simulink model "windEmulatorStep4"  (R2025b)
settings: Solver=ode4  StartTime=0.0  StopTime=inf  FixedStep=Ts  RelTol=1e-3
values from neighbouring files (symbols this model uses):
  A = 1.0    (= 1)    [initStep4.m]
  absEncoderCountsToRad = 1/2^20*2*pi    (= 5.99211245268e-06)    [initStep4.m]
  acs800CtrlStruct =     [windEmulatorBusDefs.mat]
  acs800DcBusVoltsScaling = 1    [initStep4.m]
  acs800FreqScaling = 1/100    (= 0.01)    [initStep4.m]
  acs800PowerScaling = Gen_PowerScaling    (= 14.9109)    [initStep4.m]
  acs800SignalStruct =     [windEmulatorBusDefs.mat]
  acs800SpeedNomEng = 1500    [initStep4.m]
  acs800SpeedNomFb = 20000    [initStep4.m]
  acs800SpeedScaling = 1500/20000    (= 0.075)    [initStep4.m]
  acs800TempScaling = 1/10    (= 0.1)    [initStep4.m]
  acs800TorqueNomEng = 100    [initStep4.m]
  acs800TorqueNomFb = 10000    [initStep4.m]
  acs800TorqueScaling = acs800TorqueRating/10000    (= 0.008035933)    [initStep4.m]
  acs880CtrlStruct =     [windEmulatorBusDefs.mat]
  acs880FreqScaling = 60/20000    (= 0.003)    [initStep4.m]
  acs880MotorCurrentScaling = 100/10000    (= 0.01)    [initStep4.m]
  acs880MotorVoltsScaling = 1    [initStep4.m]
  acs880PowerScaling = 100*hp2W/10000    (= 7.457)    [initStep4.m]
  acs880RatedTorque = 80.494    [initStep4.m]
  acs880RateLimFalling = -10000    [initStep4.m]
  acs880RateLimRising = 10000    [initStep4.m]
  acs880SetpointLimLower = -0.975*acs880RatedTorque    (= -78.48165)    [initStep4.m]
  acs880SetpointLimUpper = 0.975*acs880RatedTorque    (= 78.48165)    [initStep4.m]
  acs880SignalStruct =     [windEmulatorBusDefs.mat]
  acs880SpeedPILimLo = -0.975*acs880RatedTorque    (= -78.48165)    [initStep4.m]
  acs880SpeedPILimUp = 0.975*acs880RatedTorque    (= 78.48165)    [initStep4.m]
  acs880SpeedScaling = 2000/20000    (= 0.1)    [initStep4.m]
  acs880TorqueFieldbusScale = 10000    [initStep4.m]
  acs880TorqueScaling = acs880RatedTorque/acs880TorqueFieldbusScale    (= 0.0080494)    [initStep4.m]
  acs880TorqueSetpointScaling = 100    [initStep4.m]
  bar2pa = 1e5    (= 100000)    [initStep4.m]
  belowMinPGain = 1/200    (= 0.005)    [initStep4.m]
  ctrlModeTorque = logical(true)    [init.m]    (also in initStep1.m; initStep2.m; initStep3.m; initStep4.m)
  ctrlSignal1 = squeeze(hptoSignalsData.Values.ctrlSignal1.Data)    [postProcessingStep2.m]
  ctrlSignal2 = squeeze(hptoSignalsData.Values.ctrlSignal2.Data)    [postProcessingStep2.m]
  deadBandController = boolean(false)    [initStep4.m]
  deadbandTorqueSlewRate = 300    [initStep4.m]
  Dm_max = 40    [initStep4.m]
  EffMechMax = 0.93    [initStep4.m]
  EffMechMin = 0.79    [initStep4.m]
  excForce_N = squeeze(hptoCtrlData.Values.excForce_N.Data)    [postProcessingStep2.m]
  expCtrlStruct =     [windEmulatorBusDefs.mat]
  FactorEff = psi2pa*cc2m3*(1/rev2rad)    (= 0.00109733470463)    [initStep4.m]
  fromFileSpeedSlewRate = 250    [initStep4.m]
  fromFileTorqueSlewRate = 25    [initStep4.m]
  futekTorqueScale = -1/(2^31)*10/5*100    (= -9.31322574615e-08)    [initStep4.m]
  genMaxTorque = 0.8*ratedTorque    (= 64.3952)    [initStep3.m]    (also in initStep4.m = 78.48165)
  genTorqueCmd_Nm = squeeze(hptoSignalsData.Values.genTorqueCmd_Nm.Data)    [postProcessingStep2.m]
  hbmCtScale = 1/1.5    (= 0.666666666667)    [initStep4.m]
  hbmPowerStruct =     [windEmulatorBusDefs.mat]
  hptoCtrlStruct =     [windEmulatorBusDefs.mat]
  hptoSignalStruct =     [windEmulatorBusDefs.mat]
  invPowerStruct =     [windEmulatorBusDefs.mat]
  lpm2m3ps = 1/m3ps2lpm    (= 1.66666666667e-05)    [initStep4.m]
  minPressureRef_psi = 1000    [initStep4.m]
  minTorqueRef_Nm = (minPressureRef_psi*psi2pa)*(Dm_max*cc2m3*(1/rev2rad))    (= 43.8933881851)    [initStep4.m]
  motorSpeed_rpm = squeeze(acs880SignalsData.Values.motorSpeed_rpm.Data)    [postProcessingStep2.m]
  nPreDrop = 2900    [initStep4.m]
  nPreDropMin = 725    [initStep4.m]
  psi2bar = 1/bar2psi    (= 0.0689475729318)    [initStep4.m]
  radps2rpm = 60/(2*pi)    (= 9.54929658551)    [initStep2.m]    (also in initStep4.m)
  rpm2radps = 2*pi/60    (= 0.10471975512)    [initStep4.m]
  runCounter = squeeze(hptoCtrlData.Values.runCounter.Data)    [postProcessingStep2.m]
  shaftSignalStruct =     [windEmulatorBusDefs.mat]
  sidCtrlStruct =     [windEmulatorBusDefs.mat]
  sidDataCaseCounter = sidData.experimentData.count    [initStep4.m]
  sidDataSpeed_rpm = sidData.experimentData.wShaft_rpm    [initStep4.m]
  sidDataTorque_Nm = sidData.experimentData.torqueShaft_Nm    [initStep4.m]
  sidInfoStruct =     [windEmulatorBusDefs.mat]
  T = 4    [initStep4.m]
  targetOmega = 2000/60*2*pi    (= 209.439510239)    [initStep2.m]    (also in initStep3.m; initStep4.m)
  time = hptoCtrlData.Values.runCounter.Time    [postProcessingStep2.m]
  TorqueLoadMax = 75    [initStep4.m]
  Ts = 1/250    (= 0.004)    [initStep4.m]
undefined symbols (not defined in the file or in its folder): absEncoderCounts, absEncoderPosition_rad, absEncoderSpeed_rpm, absEncoderStatus1, absEncoderStatus2, absEncoderTurns, acs800Torque_Nm, acs800TorqueSetpoint_Nm, acs880SpeedSetpoint_rpm, acs880Torque_Nm, ctrlWord, dcBusVoltage_V, DiscIntNeverNeededParam, excShaftSpeed_rpm, excShaftTorque_Nm, expType, expTypeEnum, frequency_Hz, fromFileCaseCounter, genPumpFlow_lpm, genShaftSpeed_rpm, genSpeedActual, hmOutputShafTorque_Nm, motorCurrent_A, motorTorque_Nm, motorVoltage_V, pressure_bar, PressureControl, ramp, resetHilIntegrator, resetSidIntegrator, runHil, runSid, shaftPower_W, sidType, sidTypeEnum, SpeedControl, speedCtrlReset, speedRef_rpm, state, statusWord, stepCounter, temperature, torqueActual_Nm, TorqueInputControl, torqueSetpoint_Nm, torqueSetpoint_percent
libraries: slrealtimeethercatlib x118, fl_lib x26, nesl_utility x17, slrealtimeloglib x13, sh_lib x9, dspstat3 x5, simulink_extras x4, slpidlib x3, cstblocks x3, dspindex x3, simulink x2
(part 4 of 5)

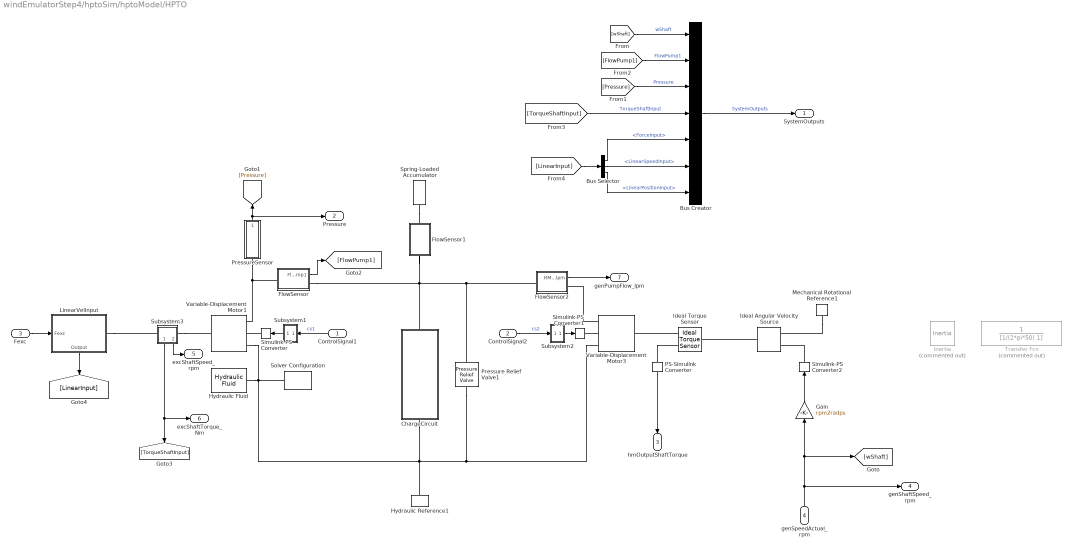
== system windEmulatorStep4/hptoSim/hptoModel/HPTO ==
  ControlSignal1 : Inport
  ControlSignal2 : Inport  Port=2
  Fexc : Inport  Port=3
  genSpeedActual_rpm : Inport  Port=4
  Bus Creator : BusCreator  Inputs=7
  Bus Selector : BusSelector  OutputSignals=ForceInput,LinearSpeedInput,LinearPositionInput
  ChargeCircuit : Subsystem
  FlowSensor : Subsystem
  FlowSensor1 : Subsystem
  FlowSensor2 : Subsystem
  Gain : Gain  Gain=rpm2radps
  Hydraulic Fluid : sh_lib/Hydraulic Utilities/Hydraulic Fluid  SelFluid=1  SysTemp=60  TrapAir=0.005  ViscDerFactor=1  range_error=1  suppress_warning=false
  Hydraulic Reference1 : fl_lib/Hydraulic/Hydraulic Elements/Hydraulic Reference
  Ideal Angular Velocity Source : fl_lib/Mechanical/Mechanical Sources/Ideal Angular Velocity Source
  Ideal Torque Sensor : fl_lib/Mechanical/Mechanical Sensors/Ideal Torque Sensor
  Inertia : fl_lib/Mechanical/Rotational Elements/Inertia  Commented=on  inertia=genShaftInertia_kgm2 kg*m^2  num_ports=foundation.enum.numPorts2.one  w_specify=off  w_priority=High  w=0 rad/s  w_nominal_specify=off  w_nominal_value=1  w_nominal_unit=rad/s  t_specify=off  t_priority=None  t=0 N*m  t_nominal_specify=off  t_nominal_value=1  t_nominal_unit=N*m
  LinearVelInput : Subsystem
      settings: PortSchema="{\"entries\":[{\"content\":{\"sides\":[{\"content\":{\"connectorIds\":[\"LConn1\"]},\"type\":\"ConnectorPlacement.EquallySpacedRectSide\",\"uuid\":\"4859a0f7-9f9b-474b-bb49-bd256c408622\"},{\"content\":{\"connectorIds\":[\"In1\"],\"side\":\"RIGHT\"},\"type\":\"ConnectorPlacement.EquallySpacedRectSide\",\"uuid\":\"5e25e59b-8f8b-4773-b6d9-951d4129523a\"},{\"content\":{\"connectorIds\":[],\"side\":\"TOP\"},\"type\":\"ConnectorPlacement.EquallySpacedRectSide\",\"uuid\":\"bae24e3d-e286-4bf4-a21b-122b1e5bc09f\"},{\"content\":{\"connectorIds\":[\"Out1\"],\"side\":\"BOTTOM\"},\"type\":\"ConnectorPlacement.EquallySpacedRectSide\",\"uuid\":\"0ce66b8b-3f3a-4f1a-9606-df56b31d9b3c\"}]},\"type\":\"ConnectorPlacement.EquallySpacedConnector\",\"uuid\":\"f87c39b6-c8d4-4afb-9096-6dab01ec5afa\"}],\"packageUris\":[\"http://schema.mathworks.com/mf0/Connector/R2020b\"],\"version\":\"1.0\"}"
  Mechanical Rotational Reference1 : fl_lib/Mechanical/Rotational Elements/Mechanical Rotational Reference
  PS-Simulink Converter : nesl_utility/PS-Simulink Converter  PhysicalDomain=network_engine_domain  SubClassName=ps_output  LeftPortType=input  RightPortType=output  PseudoPeriodic=off  Frequencies=[]  VectorFormat=1-D array  Unit=inherit  AffineConversion=off
  Pressure Relief Valve1 : sh_lib/Valves/Pressure Control Valves/Pressure Relief Valve  valve_area_spec=1  p_diff_TLU=[30.15e5 : 15e3 : 31.35e5] Pa  area_TLU=[1 : 1 : 9] .* 1e-5 m^2  area_max=(3.557e-4) m^2  pres_set=PressureValveMax psi  reg_range=ValvePreRange psi  C_d=0.7  A_leak=1e-12 m^2  lam_spec=1  B_lam=0.999  Re_cr=12  dynamic=0  tau=0.1 s  area_init=1e-12 m^2
      settings: InternalSimscapePortConfiguration="{\"Bottom\":[],\"Left\":[{\"id\":\"A\",\"label\":\"A\",\"type\":\"foundation.hydraulic.hydraulic\"}],\"Right\":[{\"id\":\"B\",\"label\":\"B\",\"type\":\"foundation.hydraulic.hydraulic\"}],\"Top\":[]}"
  PressureSensor : Subsystem
  Simulink-PS Converter : nesl_utility/Simulink-PS Converter  PhysicalDomain=network_engine_domain  SubClassName=ps_input  LeftPortType=input  RightPortType=output  PseudoPeriodic=off  Frequencies=[]  NoiseDistribution=none  NoiseParameters=[]  Unit=1  AffineConversion=off  FilteringAndDerivatives=provide  SimscapeFilterOrder=1  InputFilterTimeConstant=0.001  UdotUserProvided=0
  Simulink-PS Converter1 : nesl_utility/Simulink-PS Converter  PhysicalDomain=network_engine_domain  SubClassName=ps_input  LeftPortType=input  RightPortType=output  PseudoPeriodic=off  Frequencies=[]  NoiseDistribution=none  NoiseParameters=[]  Unit=1  AffineConversion=off  FilteringAndDerivatives=provide  SimscapeFilterOrder=1  InputFilterTimeConstant=0.001  UdotUserProvided=0
  Simulink-PS Converter2 : nesl_utility/Simulink-PS Converter  PhysicalDomain=network_engine_domain  SubClassName=ps_input  LeftPortType=input  RightPortType=output  PseudoPeriodic=off  Frequencies=[]  NoiseDistribution=none  NoiseParameters=[]  Unit=1  AffineConversion=off  FilteringAndDerivatives=provide  SimscapeFilterOrder=1  InputFilterTimeConstant=0.001  UdotUserProvided=0
  Solver Configuration : nesl_utility/Solver Configuration  PhysicalDomain=network_engine_domain  SubClassName=solver  LeftPortType=input  RightPortType=generic  Tones=[]  Harmonics=[]  SimulateNoise=off  Profile=off  UseLocalSampling=off  EnableSwitchedLinearOptims=on  FrequencyDomain=off  UseCCode=off  RelTol=0.001  AbsTol=1e-06  MinStep=1e-09  ToWorkspace=off  RevertToSquareIcSolve=off  NumHomotopyIterations=100  PhasorMode=off  PhasorModeNumHarmonics=1  ConsistencySolver=NEWTON_FTOL  IndexReductionMethod=DerivativeReplacement  DoDC=off  ResidualTolerance=1e-09  ConsistencyTolSource=GLOBAL  ConsistencyAbsTol=0.001  ConsistencyRelTol=0.001  ConsistencyTolFactor=0.001  UseLocalSolver=on  LocalSolverChoice=NE_BACKWARD_EULER_ADVANCER  ResolveIndetEquations=on  FunctionEvalNumThread=1  LocalSolverSampleTime=Ts  DoFixedCost=on  MaxNonlinIter=3  MaxModeIter=2  ComputeImpulses=off  ImpulseIterations=2  LinearAlgebra=auto  LinearAlgebraNumThread=0  EquationFormulation=NE_TIME_EF  DelaysMemoryBudget=1024  AutomaticFiltering=on  FilteringTimeConstant=0.001  PartitionStorageMethod=AS_NEEDED  PartitionMemoryBudget=1024  PartitionMethod=ROBUST  MultibodyUseLocalSolver=off  MultibodyLocalSolverChoice=ODE1  MultibodyLocalSolverSampleTime=0.001
  Spring-Loaded Accumulator : sh_lib/Accumulators/Spring-Loaded Accumulator  capacity=AccVol m^3  pr_preload=Acc_PC psi  pr_max=Acc_MaxP psi  stiff_coeff=1e10 Pa/m^3  penetr_coeff=1e10 Pa*s/m^6  flow_rate_specify=off  flow_rate_priority=None  flow_rate=5e-3 m^3/s  flow_rate_nominal_specify=off  flow_rate_nominal_value=1  flow_rate_nominal_unit=m^3/s  fluid_volume_specify=on  fluid_volume_priority=None  fluid_volume=5e-6 m^3  fluid_volume_nominal_specify=off  fluid_volume_nominal_value=1  fluid_volume_nominal_unit=m^3  fluid_pressure_specify=off  fluid_pressure_priority=None  fluid_pressure=1.01325e5 Pa  fluid_pressure_nominal_specify=off  fluid_pressure_nominal_value=1  fluid_pressure_nominal_unit=Pa
      settings: InternalSimscapePortConfiguration="{\"Bottom\":[],\"Left\":[],\"Right\":[{\"id\":\"A\",\"label\":\"A\",\"type\":\"foundation.hydraulic.hydraulic\"}],\"Top\":[]}"
  Subsystem1 : Subsystem
  Subsystem2 : Subsystem
  Subsystem3 : Subsystem
      settings: PortSchema="{\"entries\":[{\"content\":{\"sides\":[{\"content\":{\"connectorIds\":[\"LConn1\"]},\"type\":\"ConnectorPlacement.EquallySpacedRectSide\",\"uuid\":\"7d5827d5-19d2-449a-bfe5-3899d5f2f234\"},{\"content\":{\"connectorIds\":[\"RConn1\"],\"side\":\"RIGHT\"},\"type\":\"ConnectorPlacement.EquallySpacedRectSide\",\"uuid\":\"27ad7fb5-d235-43aa-a783-09c3ddbf3629\"},{\"content\":{\"connectorIds\":[],\"side\":\"TOP\"},\"type\":\"ConnectorPlacement.EquallySpacedRectSide\",\"uuid\":\"41db419c-7193-454e-a54e-cfb74ab94a84\"},{\"content\":{\"connectorIds\":[\"Out1\",\"Out2\"],\"side\":\"BOTTOM\"},\"type\":\"ConnectorPlacement.EquallySpacedRectSide\",\"uuid\":\"63d69fbc-18e5-4f7b-99db-9fcc8740eddf\"}]},\"type\":\"ConnectorPlacement.EquallySpacedConnector\",\"uuid\":\"1d29a5fa-8394-444f-93a2-8698ce035363\"}],\"packageUris\":[\"http://schema.mathworks.com/mf0/Connector/R2020b\"],\"version\":\"1.0\"}"
  Transfer Fcn : TransferFcn  Commented=on  Denominator=[1/(2*pi*50) 1]
  Variable-Displacement Motor1 : sh_lib/Pumps and Motors/Variable-Displacement Motor  mdl_type=2  stroke_max=0.005 m  D_max=Dm_max cm^3/rev  cntrl_mem_tab=[-.0075, 0, .0075] m  displ_tab=[-Dm_max, 0, Dm_max] cm^3/rev  interp_method=1  extrap_method=1  loss_spec=1  w_nominal=nShaftSpeed rpm  pr_nominal=nPreDrop psi  visc_nominal=18 cSt  dens_nominal=900 kg/m^3  efficiency_vol=EffVolNom  no_load_torque=nTorqueNoLoad N*m  torque_pressure_coeff=(1/((200-50)*1e5))*Dm_max*FactorEff*((1-EffMechMax)*nPreDrop-(1-EffMechMin)*nPreDropMin) N*m/Pa  p_diff_eff_TLU=[100000, 1000000, 2000000] Pa  omega_eff_TLU=[25, 50, 100, 200, 300, 400] rad/s  displacement_eff_TLU=[-30, -19, 19, 30] cm^3/rev  vol_eff_TLU=repmat([.816, .908, .954, .977, .981, .984; .325, .663, .831, .916, .925, .946; .137, .568, .78, .892, .893, .91], 1, 1, 4)  mech_eff_TLU=repmat([.996, .996, .996, .996, .996, .996; .988, .989, .989, .989, .989, .99; .981, .981, .982, .982, .983, .984], 1, 1, 4)  p_diff_loss_TLU=[100000, 1000000, 2000000] Pa  omega_loss_TLU=[25, 50, 100, 200, 300, 400] rad/s  displacement_loss_TLU=[-30, -19, 19, 30] cm^3/rev  vol_loss_TLU=repmat([.0282, .0253, .0241, .0235, .0291, .0325; .2596, .1271, .1017, .0917, .1216, .1142; .7874, .1901, .141, .1211, .1797, .1978] * 1e-3, 1, 1, 4) m^3/s  mech_loss_TLU=repmat([.002, .002, .002, .002, .002, .002; .06, .055, .055, .055, .055, .05; .19, .19, .18, .18, .17, .16], 1, 1, 4) N*m  pressure_threshold=1e5 Pa  omega_threshold=10 rad/s  displacement_threshold=0.0001 cm^3/rev  octant_check=0  pressure_check=0  min_valid_pressure=0 Pa  vol_eff_min=1e-3  vol_eff_max=1  mech_eff_min=1e-3  mech_eff_max=1
      settings: InternalSimscapePortConfiguration="{\"Bottom\":[],\"Left\":[{\"id\":\"A\",\"label\":\"A\",\"type\":\"foundation.hydraulic.hydraulic\"},{\"id\":\"C\",\"label\":\"C\",\"type\":\"input\"},{\"id\":\"B\",\"label\":\"B\",\"type\":\"foundation.hydraulic.hydraulic\"}],\"Right\":[{\"id\":\"S\",\"label\":\"S\",\"type\":\"foundation.mechanical.rotational.rotational\"}],\"Top\":[]}"
  Variable-Displacement Motor3 : sh_lib/Pumps and Motors/Variable-Displacement Motor  mdl_type=2  stroke_max=0.005 m  D_max=Dm_max cm^3/rev  cntrl_mem_tab=[-.0075, 0, .0075] m  displ_tab=[-Dm_max, 0, Dm_max] cm^3/rev  interp_method=1  extrap_method=1  loss_spec=1  w_nominal=nShaftSpeed rpm  pr_nominal=nPreDrop psi  visc_nominal=18 cSt  dens_nominal=900 kg/m^3  efficiency_vol=EffVolNom  no_load_torque=nTorqueNoLoad N*m  torque_pressure_coeff=(1/((200-50)*1e5))*Dm_max*FactorEff*((1-EffMechMax)*nPreDrop-(1-EffMechMin)*nPreDropMin) N*m/Pa  p_diff_eff_TLU=[100000, 1000000, 2000000] Pa  omega_eff_TLU=[25, 50, 100, 200, 300, 400] rad/s  displacement_eff_TLU=[-30, -19, 19, 30] cm^3/rev  vol_eff_TLU=repmat([.816, .908, .954, .977, .981, .984; .325, .663, .831, .916, .925, .946; .137, .568, .78, .892, .893, .91], 1, 1, 4)  mech_eff_TLU=repmat([.996, .996, .996, .996, .996, .996; .988, .989, .989, .989, .989, .99; .981, .981, .982, .982, .983, .984], 1, 1, 4)  p_diff_loss_TLU=[100000, 1000000, 2000000] Pa  omega_loss_TLU=[25, 50, 100, 200, 300, 400] rad/s  displacement_loss_TLU=[-30, -19, 19, 30] cm^3/rev  vol_loss_TLU=repmat([.0282, .0253, .0241, .0235, .0291, .0325; .2596, .1271, .1017, .0917, .1216, .1142; .7874, .1901, .141, .1211, .1797, .1978] * 1e-3, 1, 1, 4) m^3/s  mech_loss_TLU=repmat([.002, .002, .002, .002, .002, .002; .06, .055, .055, .055, .055, .05; .19, .19, .18, .18, .17, .16], 1, 1, 4) N*m  pressure_threshold=1e5 Pa  omega_threshold=10 rad/s  displacement_threshold=0.00001 cm^3/rev  octant_check=0  pressure_check=0  min_valid_pressure=0 Pa  vol_eff_min=1e-3  vol_eff_max=1  mech_eff_min=1e-3  mech_eff_max=1
      settings: InternalSimscapePortConfiguration="{\"Bottom\":[],\"Left\":[{\"id\":\"A\",\"label\":\"A\",\"type\":\"foundation.hydraulic.hydraulic\"},{\"id\":\"C\",\"label\":\"C\",\"type\":\"input\"},{\"id\":\"B\",\"label\":\"B\",\"type\":\"foundation.hydraulic.hydraulic\"}],\"Right\":[{\"id\":\"S\",\"label\":\"S\",\"type\":\"foundation.mechanical.rotational.rotational\"}],\"Top\":[]}"
  SystemOutputs : Outport
  Pressure : Outport  Port=2
  hmOutputShaftTorque : Outport  Port=3
  genShaftSpeed_rpm : Outport  Port=4
  excShaftSpeed_rpm : Outport  Port=5
  excShaftTorque_Nm : Outport  Port=6
  genPumpFlow_lpm : Outport  Port=7
  wires:
  [wShaft] -> Bus Creator/1  "wShaft"
  PressureSensor/1(Pressure) -> Pressure/1, [Pressure]
  Bus Creator/1 -> SystemOutputs/1  "SystemOutputs"
  ControlSignal1/1 -> Subsystem1/1(In1)  "cs1"
  Subsystem1/1(Out1) -> Simulink-PS Converter/1
  Subsystem2/1(Out1) -> Simulink-PS Converter1/1
  ControlSignal2/1 -> Subsystem2/1(1)  "cs2"
  FlowSensor/1(FlowPump1) -> [FlowPump1]
  [FlowPump1] -> Bus Creator/2  "FlowPump1"
  [Pressure] -> Bus Creator/3  "Pressure"
  Subsystem3/1(torque_Nm) -> excShaftTorque_Nm/1, [TorqueShaftInput]
  [TorqueShaftInput] -> Bus Creator/4  "TorqueShaftInput"
  LinearVelInput/1(Output) -> [LinearInput]
  [LinearInput] -> Bus Selector/1
  Bus Selector/2 -> Bus Creator/6  "<LinearSpeedInput>"
  Bus Selector/1 -> Bus Creator/5  "<ForceInput>"
  Bus Selector/3 -> Bus Creator/7  "<LinearPositionInput>"
  Fexc/1 -> LinearVelInput/1(Fexc)
  genSpeedActual_rpm/1 -> [wShaft], Gain/1, genShaftSpeed_rpm/1
  FlowSensor2/1(HMFlow_lpm) -> genPumpFlow_lpm/1
  Subsystem3/2(speed_rpm) -> excShaftSpeed_rpm/1
  Gain/1 -> Simulink-PS Converter2/1
  PS-Simulink Converter/1 -> hmOutputShaftTorque/1
  connections:
  FlowSensor1/LConn1 -- FlowSensor/RConn1 -- Pressure Relief Valve1/LConn1 -- FlowSensor2/LConn1 -- ChargeCircuit/LConn1
  PressureSensor/LConn1 -- FlowSensor/LConn1 -- Variable-Displacement Motor1/LConn1
  Variable-Displacement Motor3/LConn2 -- Simulink-PS Converter1/RConn1
  Simulink-PS Converter/RConn1 -- Variable-Displacement Motor1/LConn2
  Spring-Loaded Accumulator/RConn1 -- FlowSensor1/RConn1
  Variable-Displacement Motor3/LConn1 -- FlowSensor2/RConn1
  Subsystem3/RConn1 -- Variable-Displacement Motor1/RConn1
  LinearVelInput/LConn1 -- Subsystem3/LConn1
  Variable-Displacement Motor1/LConn3 -- Pressure Relief Valve1/RConn1 -- Variable-Displacement Motor3/LConn3 -- Hydraulic Reference1/LConn1 -- ChargeCircuit/RConn1 -- Solver Configuration/RConn1 -- Hydraulic Fluid/RConn1
  Simulink-PS Converter2/RConn1 -- Ideal Angular Velocity Source/RConn1
  Mechanical Rotational Reference1/LConn1 -- Ideal Angular Velocity Source/RConn2
  Ideal Torque Sensor/RConn1 -- Variable-Displacement Motor3/RConn1
  PS-Simulink Converter/LConn1 -- Ideal Torque Sensor/RConn2
  Ideal Angular Velocity Source/LConn1 -- Ideal Torque Sensor/LConn1

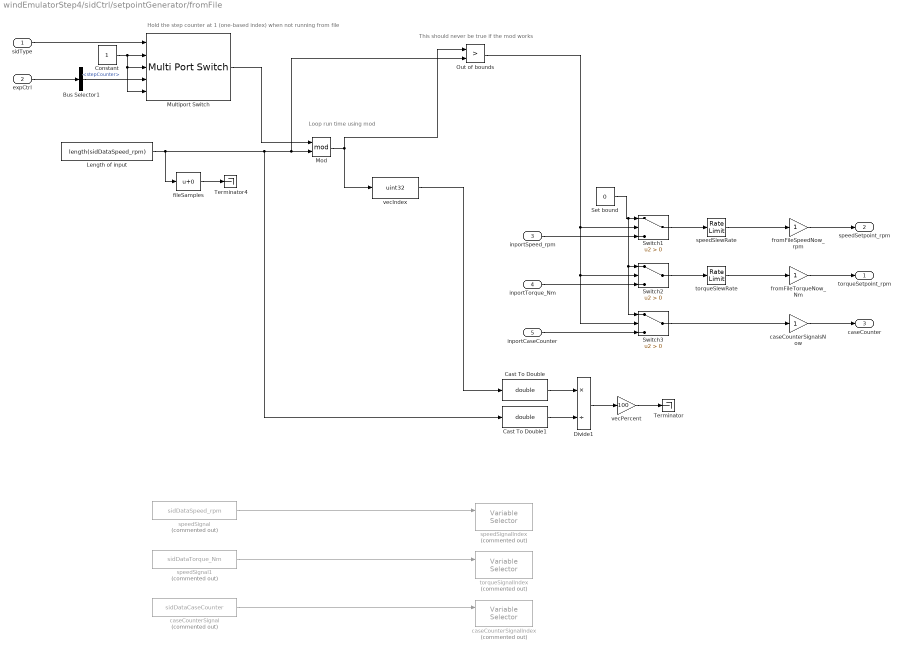
== system windEmulatorStep4/sidCtrl/setpointGenerator/fromFile ==
  note: Hold the step counter at 1 (one-based index) when not running from file
  note: This should never be true if the mod works
  note: Loop run time using mod
  sidType : Inport  OutDataTypeStr=Enum: sidTypeEnum
  expCtrl : Inport  Port=2  OutDataTypeStr=Bus: expCtrlBus
  inportSpeed_rpm : Inport  Port=3
  inportTorque_Nm : Inport  Port=4
  inportCaseCounter : Inport  Port=5
  Bus Selector1 : BusSelector  OutputSignals=stepCounter
  Cast To Double : DataTypeConversion  OutDataTypeStr=double  SaturateOnIntegerOverflow=off  RndMeth=Floor
  Cast To Double1 : DataTypeConversion  OutDataTypeStr=double  SaturateOnIntegerOverflow=off  RndMeth=Floor
  Constant : Constant  OutDataTypeStr=uint32
  Divide1 : Product  Inputs=*/
  Length of input : Constant  Value=length(sidDataSpeed_rpm)  OutDataTypeStr=uint32
  Mod : Math  Operator=mod
  Multiport Switch : MultiPortSwitch  DataPortOrder=Specify indices  DataPortIndices={sidTypeEnum.off,sidTypeEnum.manual,sidTypeEnum.fromFile}  DataPortForDefault=Additional data port  SaturateOnIntegerOverflow=off  InputSameDT=off
  Out of bounds : RelationalOperator  Operator=>  OutDataTypeStr=boolean  RndMeth=Simplest  InputSameDT=off
  Set bound : Constant  Value=0
  Switch1 : Switch  Criteria=u2 > Threshold  SaturateOnIntegerOverflow=off  InputSameDT=off
  Switch2 : Switch  Criteria=u2 > Threshold  SaturateOnIntegerOverflow=off  InputSameDT=off
  Switch3 : Switch  Criteria=u2 > Threshold  SaturateOnIntegerOverflow=off  InputSameDT=off
  Terminator : Terminator
  Terminator4 : Terminator
  caseCounterSignal : Constant  Commented=on  Value=sidDataCaseCounter
  caseCounterSignalIndex : dspindex/Variable Selector  Commented=on  NumInputs=1  rowsOrCols=Columns  IdxMode=Variable  Elements=[1 3]  ZerOneIdxMode=One-based  errmode=Clip and Warn  FillMode=on  FillValues=0
  caseCounterSignalsNow : Gain
  fileSamples : Bias  SaturateOnIntegerOverflow=off
  fromFileSpeedNow_rpm : Gain
  fromFileTorqueNow_Nm : Gain
  speedSignal : Constant  Commented=on  Value=sidDataSpeed_rpm
  speedSignal1 : Constant  Commented=on  Value=sidDataTorque_Nm
  speedSignalIndex : dspindex/Variable Selector  Commented=on  NumInputs=1  rowsOrCols=Columns  IdxMode=Variable  Elements=[1 3]  ZerOneIdxMode=One-based  errmode=Clip and Warn  FillMode=on  FillValues=0
  speedSlewRate : RateLimiter  RisingSlewLimit=fromFileSpeedSlewRate  FallingSlewLimit=-fromFileSpeedSlewRate  SampleTimeMode=inherited
  torqueSignalIndex : dspindex/Variable Selector  Commented=on  NumInputs=1  rowsOrCols=Columns  IdxMode=Variable  Elements=[1 3]  ZerOneIdxMode=One-based  errmode=Clip and Warn  FillMode=on  FillValues=0
  torqueSlewRate : RateLimiter  RisingSlewLimit=fromFileTorqueSlewRate  FallingSlewLimit=-fromFileTorqueSlewRate  SampleTimeMode=inherited
  vecIndex : DataTypeConversion  OutDataTypeStr=uint32  SaturateOnIntegerOverflow=off  RndMeth=Floor
  vecPercent : Gain  Gain=100
  torqueSetpoint_rpm : Outport
  speedSetpoint_rpm : Outport  Port=2
  caseCounter : Outport  Port=3
  wires:
  vecPercent/1 -> Terminator/1
  Cast To Double/1 -> Divide1/1
  Length of input/1 -> Cast To Double1/1, Out of bounds/2, Mod/2, fileSamples/1
  fromFileTorqueNow_Nm/1 -> torqueSetpoint_rpm/1
  speedSignal/1 -> speedSignalIndex/1
  Out of bounds/1 -> Switch3/2, Switch2/2, Switch1/2
  torqueSlewRate/1 -> fromFileTorqueNow_Nm/1
  caseCounterSignal/1 -> caseCounterSignalIndex/1
  Switch2/1 -> torqueSlewRate/1
  speedSlewRate/1 -> fromFileSpeedNow_rpm/1
  vecIndex/1 -> Cast To Double/1
  Set bound/1 -> Switch2/1, Switch3/1, Switch1/1
  Switch1/1 -> speedSlewRate/1
  Mod/1 -> vecIndex/1, Out of bounds/1
  fileSamples/1 -> Terminator4/1
  Divide1/1 -> vecPercent/1
  caseCounterSignalsNow/1 -> caseCounter/1
  Switch3/1 -> caseCounterSignalsNow/1
  fromFileSpeedNow_rpm/1 -> speedSetpoint_rpm/1
  Cast To Double1/1 -> Divide1/2
  expCtrl/1 -> Bus Selector1/1
  speedSignal1/1 -> torqueSignalIndex/1
  sidType/1 -> Multiport Switch/1
  Bus Selector1/1 -> Multiport Switch/4  "<stepCounter>"
  Multiport Switch/1 -> Mod/1
  Constant/1 -> Multiport Switch/5, Multiport Switch/3, Multiport Switch/2
  inportSpeed_rpm/1 -> Switch1/3
  inportTorque_Nm/1 -> Switch2/3
  inportCaseCounter/1 -> Switch3/3

== system windEmulatorStep4/hptoSim/hptoModel/ControlAlgorithm/ForceToTorque ==
  ActualSignals : Inport
  Bus Selector : BusSelector  OutputSignals=LinearSpeedInput,LinearPositionInput
  Constant2 : Constant  Value=(A*2*pi/T)/targetOmega
  DesiredForce : Subsystem
  Gain : Gain  Gain=-1
  Product2 : Product
  TorqueD : Outport
  wires:
  ActualSignals/1 -> Bus Selector/1
  Product2/1 -> Gain/1
  Constant2/1 -> Product2/2
  Bus Selector/1 -> DesiredForce/1(<LinearSpeedInput>)  "<LinearSpeedInput>"
  Bus Selector/2 -> DesiredForce/2(<LinearPositionInput>)  "<LinearPositionInput>"
  DesiredForce/1(ForceD) -> Product2/1
  Gain/1 -> TorqueD/1

== system windEmulatorStep4/hptoSim/hptoModel/ControlAlgorithm/PressureAbovePmin ==
  ActualSignals : Inport
  RefValues : Inport  Port=2
  SpeedControllerReset : Inport  Port=3
  Bus Selector : BusSelector  OutputSignals=TorqueShaftInput,Pressure,wShaft
  Bus Selector1 : BusSelector  OutputSignals=TorqueInputRef,PressureRef,SheftSpeedRef
  PressureControl1 : Subsystem
  SpeedControl1 : Subsystem
  Terminator1 : Terminator
  TorqueControl1 : Subsystem
  ControlSignal1 : Outport
  ControlSignal2 : Outport  Port=2
  ControlTorqueLoad : Outport  Port=3
  wires:
  ActualSignals/1 -> Bus Selector/1
  TorqueControl1/1(ControlSignal1) -> ControlSignal1/1
  Bus Selector/3 -> SpeedControl1/1(ShaftSpeedMotor)  "<wShaft>"
  RefValues/1 -> Bus Selector1/1
  Bus Selector1/1 -> TorqueControl1/1(TorqueRef)  "<TorqueInputRef>"
  Bus Selector1/3 -> SpeedControl1/2(ShaftSpeedRef)  "<SheftSpeedRef>"
  PressureControl1/1(ControlSignal2) -> ControlSignal2/1
  Bus Selector/2 -> PressureControl1/1(ActualPressure)  "<Pressure>"
  Bus Selector/1 -> Terminator1/1  "<TorqueShaftInput>"
  Bus Selector1/2 -> PressureControl1/2(PressureRef)  "<PressureRef>"
  SpeedControl1/1(ContolTorque) -> ControlTorqueLoad/1
  SpeedControllerReset/1 -> SpeedControl1/3(SpeedControllerReset)

== system windEmulatorStep4/hptoSim/hptoModel/ControlAlgorithm/PressureBelowPmin ==
  ActualSignals : Inport
  RefValues : Inport  Port=2
  SpeedControllerReset : Inport  Port=3
  Bus Selector : BusSelector  OutputSignals=TorqueShaftInput,Pressure,wShaft
  Bus Selector1 : BusSelector  OutputSignals=TorqueInputRef,PressureRef,SheftSpeedRef
  PressureControl1 : Subsystem
  SpeedControl1 : Subsystem
  TorqueControl1 : Subsystem
  ControlSignal1 : Outport
  ControlSignal2 : Outport  Port=2
  ControlTorqueLoad : Outport  Port=3
  wires:
  ActualSignals/1 -> Bus Selector/1
  Bus Selector/1 -> TorqueControl1/1(ActualTorqueInput)  "<TorqueShaftInput>"
  TorqueControl1/1(ControlSignal1) -> ControlSignal1/1
  PressureControl1/1(ControlSignal2) -> ControlSignal2/1
  Bus Selector/2 -> TorqueControl1/3(Pressure), PressureControl1/1(ActualPressure)  "<Pressure>"
  Bus Selector/3 -> SpeedControl1/1(ShaftSpeedMotor)  "<wShaft>"
  SpeedControl1/1(ContolTorque) -> ControlTorqueLoad/1
  RefValues/1 -> Bus Selector1/1
  Bus Selector1/1 -> TorqueControl1/2(TorqueRef)  "<TorqueInputRef>"
  Bus Selector1/2 -> PressureControl1/2(PressureRef)  "<PressureRef>"
  Bus Selector1/3 -> SpeedControl1/2(ShaftSpeedRef)  "<SheftSpeedRef>"
  SpeedControllerReset/1 -> SpeedControl1/3(SpeedControllerReset)

== system windEmulatorStep4/hptoSim/hptoModel/HPTO/ChargeCircuit ==
  note: Pressure compensated charge pump
  Check Valve1 : sh_lib/Valves/Directional Valves/Check Valve  area_max=1e-2 m^2  pres_crack=2 bar  pres_max=4 bar  C_d=0.7  A_leak=1e-12 m^2  lam_spec=1  B_lam=0.999  Re_cr=12  dynamic=0  tau=0.1 s  area_init=1e-12 m^2
      settings: InternalSimscapePortConfiguration="{\"Bottom\":[],\"Left\":[{\"id\":\"A\",\"label\":\"A\",\"type\":\"foundation.hydraulic.hydraulic\"}],\"Right\":[{\"id\":\"B\",\"label\":\"B\",\"type\":\"foundation.hydraulic.hydraulic\"}],\"Top\":[]}"
  Constant1 : Constant  Value=2000*rpm2radps
  Gas-Charged Accumulator2 : sh_lib/Accumulators/Gas-Charged Accumulator  capacity=5e-3 m^3  dead_volume=4e-5 m^3  pr_preload=100 psi  k_sh=1.4  stiff_coeff=1e10 Pa/m^3  penetr_coeff=1e10 Pa*s/m^6  flow_rate_specify=off  flow_rate_priority=None  flow_rate=5e-3 m^3/s  flow_rate_nominal_specify=off  flow_rate_nominal_value=1  flow_rate_nominal_unit=m^3/s  liquid_volume_specify=on  liquid_volume_priority=High  liquid_volume=4.9e-3 m^3  liquid_volume_nominal_specify=off  liquid_volume_nominal_value=1  liquid_volume_nominal_unit=m^3  liquid_pressure_specify=on  liquid_pressure_priority=High  liquid_pressure=400 psi  liquid_pressure_nominal_specify=off  liquid_pressure_nominal_value=1  liquid_pressure_nominal_unit=Pa
      settings: InternalSimscapePortConfiguration="{\"Bottom\":[],\"Left\":[],\"Right\":[{\"id\":\"A\",\"label\":\"A\",\"type\":\"foundation.hydraulic.hydraulic\"}],\"Top\":[]}"
  Ideal Angular Velocity Source : fl_lib/Mechanical/Mechanical Sources/Ideal Angular Velocity Source
  Mechanical Rotational Reference : fl_lib/Mechanical/Rotational Elements/Mechanical Rotational Reference
  Pressure Relief Valve2 : sh_lib/Valves/Pressure Control Valves/Pressure Relief Valve  valve_area_spec=1  p_diff_TLU=[30.15e5 : 15e3 : 31.35e5] Pa  area_TLU=[1 : 1 : 9] .* 1e-5 m^2  area_max=1e-4 m^2  pres_set=30 bar  reg_range=1 bar  C_d=0.7  A_leak=1e-12 m^2  lam_spec=1  B_lam=0.999  Re_cr=12  dynamic=0  tau=0.1 s  area_init=1e-12 m^2
      settings: InternalSimscapePortConfiguration="{\"Bottom\":[],\"Left\":[{\"id\":\"A\",\"label\":\"A\",\"type\":\"foundation.hydraulic.hydraulic\"}],\"Right\":[{\"id\":\"B\",\"label\":\"B\",\"type\":\"foundation.hydraulic.hydraulic\"}],\"Top\":[]}"
  Rate Limiter : RateLimiter  RisingSlewLimit=200  FallingSlewLimit=-200  SampleTimeMode=inherited
  Simulink-PS Converter1 : nesl_utility/Simulink-PS Converter  PhysicalDomain=network_engine_domain  SubClassName=ps_input  LeftPortType=input  RightPortType=output  PseudoPeriodic=off  Frequencies=[]  NoiseDistribution=none  NoiseParameters=[]  Unit=1  AffineConversion=off  FilteringAndDerivatives=provide  SimscapeFilterOrder=1  InputFilterTimeConstant=0.001  UdotUserProvided=0
  Variable-Displacement Pressure-Compensated Pump1 : sh_lib/Pumps and Motors/Variable-Displacement Pressure-Compensated Pump  D_max=0.2 l/rev  pr_set=20 bar  pr_reg=1 bar  efficiency_vol=0.85  efficiency_tot=0.75  pr_nominal=20 bar  w_nominal=1800 rpm  visc_nominal=18 cSt  dens_nominal=950 kg/m^3
      settings: InternalSimscapePortConfiguration="{\"Bottom\":[],\"Left\":[{\"id\":\"S\",\"label\":\"S\",\"type\":\"foundation.mechanical.rotational.rotational\"}],\"Right\":[{\"id\":\"P\",\"label\":\"P\",\"type\":\"foundation.hydraulic.hydraulic\"},{\"id\":\"T\",\"label\":\"T\",\"type\":\"foundation.hydraulic.hydraulic\"}],\"Top\":[]}"
  Conn1 : PMIOPort  Side=Left
  Conn2 : PMIOPort  Port=2  Side=Right
  wires:
  Rate Limiter/1 -> Simulink-PS Converter1/1
  Constant1/1 -> Rate Limiter/1
  connections:
  Variable-Displacement Pressure-Compensated Pump1/RConn2 -- Pressure Relief Valve2/RConn1 -- Conn2/RConn1
  Variable-Displacement Pressure-Compensated Pump1/RConn1 -- Gas-Charged Accumulator2/RConn1 -- Check Valve1/LConn1 -- Pressure Relief Valve2/LConn1
  Simulink-PS Converter1/RConn1 -- Ideal Angular Velocity Source/RConn1
  Ideal Angular Velocity Source/RConn2 -- Mechanical Rotational Reference/LConn1
  Variable-Displacement Pressure-Compensated Pump1/LConn1 -- Ideal Angular Velocity Source/LConn1
  Conn1/RConn1 -- Check Valve1/RConn1

== system windEmulatorStep4/hptoSim/hptoModel/HPTO/FlowSensor ==
  Hydraulic Flow Rate Sensor : fl_lib/Hydraulic/Hydraulic Sensors/Hydraulic Flow Rate Sensor
  PS Terminator : fl_lib/Physical Signals/Sinks/PS Terminator
  PS-Simulink Converter : nesl_utility/PS-Simulink Converter  PhysicalDomain=network_engine_domain  SubClassName=ps_output  LeftPortType=input  RightPortType=output  PseudoPeriodic=off  Frequencies=[]  VectorFormat=1-D array  Unit=inherit  AffineConversion=off
  Scope : Scope
  m3toL : Gain  Gain=1000*60
  Qin : PMIOPort  Side=Left
  Qout : PMIOPort  Port=2  Side=Right
  FlowPump1 : Outport
  wires:
  PS-Simulink Converter/1 -> m3toL/1, Scope/1
  m3toL/1 -> FlowPump1/1  "FlowPump1"
  connections:
  PS-Simulink Converter/LConn1 -- Hydraulic Flow Rate Sensor/RConn1
  Hydraulic Flow Rate Sensor/RConn2 -- Qout/RConn1
  PS Terminator/LConn1 -- Hydraulic Flow Rate Sensor/RConn3
  Hydraulic Flow Rate Sensor/LConn1 -- Qin/RConn1

== system windEmulatorStep4/hptoSim/hptoModel/HPTO/FlowSensor1 ==
  Gain : Gain  Gain=1000*60
  Hydraulic Flow Rate Sensor : fl_lib/Hydraulic/Hydraulic Sensors/Hydraulic Flow Rate Sensor
  PS Terminator : fl_lib/Physical Signals/Sinks/PS Terminator
  PS-Simulink Converter : nesl_utility/PS-Simulink Converter  PhysicalDomain=network_engine_domain  SubClassName=ps_output  LeftPortType=input  RightPortType=output  PseudoPeriodic=off  Frequencies=[]  VectorFormat=1-D array  Unit=inherit  AffineConversion=off
  Scope : Scope
  Qin : PMIOPort  Side=Left
  Qout : PMIOPort  Port=2  Side=Right
  wires:
  PS-Simulink Converter/1 -> Gain/1
  Gain/1 -> Scope/1  "FlowAccumulator"
  connections:
  PS-Simulink Converter/LConn1 -- Hydraulic Flow Rate Sensor/RConn1
  Hydraulic Flow Rate Sensor/RConn2 -- Qout/RConn1
  PS Terminator/LConn1 -- Hydraulic Flow Rate Sensor/RConn3
  Hydraulic Flow Rate Sensor/LConn1 -- Qin/RConn1

== system windEmulatorStep4/hptoSim/hptoModel/HPTO/FlowSensor2 ==
  Gain : Gain  Gain=1000*60
  Hydraulic Flow Rate Sensor : fl_lib/Hydraulic/Hydraulic Sensors/Hydraulic Flow Rate Sensor
  PS Terminator : fl_lib/Physical Signals/Sinks/PS Terminator
  PS-Simulink Converter : nesl_utility/PS-Simulink Converter  PhysicalDomain=network_engine_domain  SubClassName=ps_output  LeftPortType=input  RightPortType=output  PseudoPeriodic=off  Frequencies=[]  VectorFormat=1-D array  Unit=inherit  AffineConversion=off
  Qin : PMIOPort  Side=Left
  Qout : PMIOPort  Port=2  Side=Right
  HMFlow_lpm : Outport
  wires:
  PS-Simulink Converter/1 -> Gain/1
  Gain/1 -> HMFlow_lpm/1  "FlowMotor1"
  connections:
  PS-Simulink Converter/LConn1 -- Hydraulic Flow Rate Sensor/RConn1
  Hydraulic Flow Rate Sensor/RConn2 -- Qout/RConn1
  PS Terminator/LConn1 -- Hydraulic Flow Rate Sensor/RConn3
  Hydraulic Flow Rate Sensor/LConn1 -- Qin/RConn1

== system windEmulatorStep4/hptoSim/hptoModel/HPTO/LinearVelInput ==
  Fexc : Inport
  Ideal Force Sensor1 : fl_lib/Mechanical/Mechanical Sensors/Ideal Force Sensor
  PS-Simulink Converter : nesl_utility/PS-Simulink Converter  PhysicalDomain=network_engine_domain  SubClassName=ps_output  LeftPortType=input  RightPortType=output  PseudoPeriodic=off  Frequencies=[]  VectorFormat=1-D array  Unit=inherit  AffineConversion=off
  Subsystem : Subsystem
      settings: PortSchema="{\"entries\":[{\"content\":{\"sides\":[{\"content\":{\"connectorIds\":[\"LConn1\"]},\"type\":\"ConnectorPlacement.EquallySpacedRectSide\",\"uuid\":\"215b7bca-b171-42a0-8110-3ac7d91926b2\"},{\"content\":{\"connectorIds\":[\"RConn1\"],\"side\":\"RIGHT\"},\"type\":\"ConnectorPlacement.EquallySpacedRectSide\",\"uuid\":\"231e152d-bce3-44d9-a550-7c1231ef5d98\"},{\"content\":{\"connectorIds\":[],\"side\":\"TOP\"},\"type\":\"ConnectorPlacement.EquallySpacedRectSide\",\"uuid\":\"bc851d42-4603-42fa-9c49-ea05891b2ab9\"},{\"content\":{\"connectorIds\":[\"Out1\"],\"side\":\"BOTTOM\"},\"type\":\"ConnectorPlacement.EquallySpacedRectSide\",\"uuid\":\"67c0fa27-8a6c-4f46-81b7-2dea8cbe6936\"}]},\"type\":\"ConnectorPlacement.EquallySpacedConnector\",\"uuid\":\"7442d2b0-500a-4e34-82e4-4fa764ec5830\"}],\"packageUris\":[\"http://schema.mathworks.com/mf0/Connector/R2020b\"],\"version\":\"1.0\"}"
  WavebotModel : Subsystem
  Wheel and Axle : fl_lib/Mechanical/Mechanisms/Wheel and Axle  R=(A*2*pi/T)/targetOmega m  or=1  t_specify=off  t_priority=None  t=0 N*m  t_nominal_specify=off  t_nominal_value=1  t_nominal_unit=N*m  f_specify=off  f_priority=None  f=0 N  f_nominal_specify=off  f_nominal_value=1  f_nominal_unit=N
  Shaft : PMIOPort  Side=Left
  Output : Outport
  wires:
  Subsystem/1(LinearInput) -> Output/1
  PS-Simulink Converter/1 -> WavebotModel/1(PTOForce)
  Fexc/1 -> WavebotModel/2(Fexc)
  connections:
  PS-Simulink Converter/LConn1 -- Ideal Force Sensor1/RConn2
  WavebotModel/RConn1 -- Ideal Force Sensor1/RConn1
  Subsystem/LConn1 -- Ideal Force Sensor1/LConn1
  Wheel and Axle/RConn1 -- Subsystem/RConn1
  Wheel and Axle/LConn1 -- Shaft/RConn1

== system windEmulatorStep4/hptoSim/hptoModel/HPTO/PressureSensor ==
  Gain : Gain  Gain=1/6894.75
  Hydraulic Pressure Sensor : fl_lib/Hydraulic/Hydraulic Sensors/Hydraulic Pressure Sensor
  Hydraulic Reference2 : fl_lib/Hydraulic/Hydraulic Elements/Hydraulic Reference
  PS-Simulink Converter : nesl_utility/PS-Simulink Converter  PhysicalDomain=network_engine_domain  SubClassName=ps_output  LeftPortType=input  RightPortType=output  PseudoPeriodic=off  Frequencies=[]  VectorFormat=1-D array  Unit=inherit  AffineConversion=off
  Scope : Scope
  P : PMIOPort  Side=Left
  Pressure : Outport
  wires:
  PS-Simulink Converter/1 -> Gain/1
  Gain/1 -> Pressure/1, Scope/1  "Pressure"
  connections:
  PS-Simulink Converter/LConn1 -- Hydraulic Pressure Sensor/RConn2
  Hydraulic Reference2/LConn1 -- Hydraulic Pressure Sensor/RConn1
  Hydraulic Pressure Sensor/LConn1 -- P/RConn1

== system windEmulatorStep4/hptoSim/hptoModel/HPTO/Subsystem1 ==
  In1 : Inport
  Gain : Gain  Gain=0.0075
  LTI System2 : cstblocks/LTI System  sys=tf(100*2*pi,[1 200*pi])  IC=[]  PadeOrder=0
  Out1 : Outport
  wires:
  LTI System2/1 -> Gain/1
  In1/1 -> LTI System2/1
  Gain/1 -> Out1/1

== system windEmulatorStep4/hptoSim/hptoModel/HPTO/Subsystem2 ==
  1 : Inport
  Gain : Gain  Gain=0.0075
  LTI System2 : cstblocks/LTI System  sys=tf(100*2*pi,[1 200*pi])  IC=[]  PadeOrder=0
  Out1 : Outport
  wires:
  LTI System2/1 -> Gain/1
  1/1 -> LTI System2/1
  Gain/1 -> Out1/1

== system windEmulatorStep4/hptoSim/hptoModel/HPTO/Subsystem3 ==
  Gain : Gain  Gain=radps2rpm
  Ideal Rotational Motion Sensor : fl_lib/Mechanical/Mechanical Sensors/Ideal Rotational Motion Sensor  reference=foundation.enum.MeasurementReference.difference  acceleration_port=false  velocity_port=true  position_port=true  wrap_angle=simscape.enum.onoff.off  offset=0 rad
  Ideal Torque Sensor : fl_lib/Mechanical/Mechanical Sensors/Ideal Torque Sensor
  Mechanical Rotational Reference : fl_lib/Mechanical/Rotational Elements/Mechanical Rotational Reference
  PS Terminator : fl_lib/Physical Signals/Sinks/PS Terminator
  PS-Simulink Converter : nesl_utility/PS-Simulink Converter  PhysicalDomain=network_engine_domain  SubClassName=ps_output  LeftPortType=input  RightPortType=output  PseudoPeriodic=off  Frequencies=[]  VectorFormat=1-D array  Unit=inherit  AffineConversion=off
  PS-Simulink Converter1 : nesl_utility/PS-Simulink Converter  PhysicalDomain=network_engine_domain  SubClassName=ps_output  LeftPortType=input  RightPortType=output  PseudoPeriodic=off  Frequencies=[]  VectorFormat=1-D array  Unit=inherit  AffineConversion=off
  1 : PMIOPort  Side=Left
  2 : PMIOPort  Port=2  Side=Right
  torque_Nm : Outport
  speed_rpm : Outport  Port=2
  wires:
  PS-Simulink Converter/1 -> torque_Nm/1  "TorqueInput"
  PS-Simulink Converter1/1 -> Gain/1
  Gain/1 -> speed_rpm/1  "ShaftSpeedPump"
  connections:
  Ideal Rotational Motion Sensor/LConn1 -- Ideal Torque Sensor/LConn1 -- 1/RConn1
  Mechanical Rotational Reference/LConn1 -- Ideal Rotational Motion Sensor/RConn1
  PS Terminator/LConn1 -- Ideal Rotational Motion Sensor/RConn3
  PS-Simulink Converter1/LConn1 -- Ideal Rotational Motion Sensor/RConn2
  Ideal Torque Sensor/RConn1 -- 2/RConn1
  PS-Simulink Converter/LConn1 -- Ideal Torque Sensor/RConn2

== system windEmulatorStep4/hptoSim/hptoModel/ControlAlgorithm/ForceToTorque/DesiredForce ==
  <LinearSpeedInput> : Inport
  <LinearPositionInput> : Inport  Port=2
  Add : Sum
  Product : Product
  Product1 : Product
  kDamping : Constant  Value=0
  kDampingNow : Gain
  kSpring : Constant  Value=0
  kSpringNow : Gain
  ForceD : Outport
  wires:
  Add/1 -> ForceD/1  "ForceD"
  kSpring/1 -> kSpringNow/1
  kDamping/1 -> kDampingNow/1
  Product1/1 -> Add/2
  Product/1 -> Add/1
  <LinearPositionInput>/1 -> Product1/1
  <LinearSpeedInput>/1 -> Product/2
  kDampingNow/1 -> Product/1
  kSpringNow/1 -> Product1/2

== system windEmulatorStep4/hptoSim/hptoModel/ControlAlgorithm/PressureAbovePmin/PressureControl1 ==
  ActualPressure : Inport
  PressureRef : Inport  Port=2
  Add : Sum
  Discrete-Time Integrator : DiscreteIntegrator  SampleTime=-1  ICPrevOutput=DiscIntNeverNeededParam  ICPrevScaledInput=DiscIntNeverNeededParam
  Gain : Gain  Gain=PressureControl.PG
  Gain1 : Gain  Gain=PressureControl.IG
  Saturation : Saturate  UpperLimit=1  LowerLimit=-1
  Sum : Sum  Inputs=|-+
  ControlSignal2 : Outport
  wires:
  PressureRef/1 -> Sum/1
  ActualPressure/1 -> Sum/2
  Sum/1 -> Discrete-Time Integrator/1, Gain/1
  Gain/1 -> Add/1
  Discrete-Time Integrator/1 -> Gain1/1
  Gain1/1 -> Add/2
  Saturation/1 -> ControlSignal2/1
  Add/1 -> Saturation/1

== system windEmulatorStep4/hptoSim/hptoModel/ControlAlgorithm/PressureAbovePmin/SpeedControl1 ==
  ShaftSpeedMotor : Inport
  ShaftSpeedRef : Inport  Port=2
  SpeedControllerReset : Inport  Port=3
  DeadBandController : Constant  Value=deadBandController  OutDataTypeStr=boolean
  Rate Limiter : RateLimiter  RisingSlewLimit=deadbandTorqueSlewRate  FallingSlewLimit=-deadbandTorqueSlewRate  SampleTimeMode=inherited
  Rate Limiter1 : RateLimiter  RisingSlewLimit=50  FallingSlewLimit=-50  SampleTimeMode=inherited
  Subsystem : Subsystem
  Subsystem1 : Subsystem
  Switch : Switch  Criteria=u2 > Threshold  SaturateOnIntegerOverflow=off  InputSameDT=off
  shaftSpeedRefMin : Constant  Value=0
  ContolTorque : Outport
  wires:
  ShaftSpeedRef/1 -> Subsystem/1(shaftSpeedRef), Subsystem1/2(ShaftSpeedRefMax)
  ShaftSpeedMotor/1 -> Subsystem1/1(ShaftSpeed), Subsystem/2(shaftSpeedMotor)
  SpeedControllerReset/1 -> Subsystem/3(Reset)
  shaftSpeedRefMin/1 -> Rate Limiter1/1
  Switch/1 -> ContolTorque/1
  DeadBandController/1 -> Switch/2
  Subsystem1/1(ControlTorque_Nm) -> Rate Limiter/1
  Subsystem/1(ContolTorque_Nm) -> Switch/3
  Rate Limiter/1 -> Switch/1
  Rate Limiter1/1 -> Subsystem1/3(ShaftSpeedRefMin)

== system windEmulatorStep4/hptoSim/hptoModel/ControlAlgorithm/PressureAbovePmin/TorqueControl1 ==
  TorqueRef : Inport
  Constant : Constant  Value=-1
  Constant1 : Constant
  Switch : Switch  SaturateOnIntegerOverflow=off  InputSameDT=off
  ControlSignal1 : Outport
  wires:
  TorqueRef/1 -> Switch/2
  Constant/1 -> Switch/1
  Constant1/1 -> Switch/3
  Switch/1 -> ControlSignal1/1

== system windEmulatorStep4/hptoSim/hptoModel/ControlAlgorithm/PressureBelowPmin/PressureControl1 ==
  ActualPressure : Inport
  PressureRef : Inport  Port=2
  Add : Sum
  Discrete-Time Integrator : DiscreteIntegrator  SampleTime=-1  ICPrevOutput=DiscIntNeverNeededParam  ICPrevScaledInput=DiscIntNeverNeededParam
  Gain : Gain  Gain=PressureControl.PG
  Gain1 : Gain  Gain=PressureControl.IG
  Saturation : Saturate  UpperLimit=1  LowerLimit=-1
  Sum : Sum  Inputs=|-+
  ControlSignal2 : Outport
  wires:
  PressureRef/1 -> Sum/1
  ActualPressure/1 -> Sum/2
  Sum/1 -> Discrete-Time Integrator/1, Gain/1
  Gain/1 -> Add/1
  Discrete-Time Integrator/1 -> Gain1/1
  Gain1/1 -> Add/2
  Saturation/1 -> ControlSignal2/1
  Add/1 -> Saturation/1

== system windEmulatorStep4/hptoSim/hptoModel/ControlAlgorithm/PressureBelowPmin/SpeedControl1 ==
  ShaftSpeedMotor : Inport
  ShaftSpeedRef : Inport  Port=2
  SpeedControllerReset : Inport  Port=3
  DeadBandController : Constant  Value=deadBandController
  Rate Limiter : RateLimiter  RisingSlewLimit=deadbandTorqueSlewRate  FallingSlewLimit=-deadbandTorqueSlewRate  SampleTimeMode=inherited
  Rate Limiter1 : RateLimiter  RisingSlewLimit=50  FallingSlewLimit=-50  SampleTimeMode=inherited
  Subsystem : Subsystem
  Subsystem1 : Subsystem
  Switch : Switch  Criteria=u2 > Threshold  SaturateOnIntegerOverflow=off  InputSameDT=off
  shaftSpeedRefMin : Constant  Value=0
  ContolTorque : Outport
  wires:
  ShaftSpeedRef/1 -> Subsystem/1(shaftSpeedRef), Subsystem1/2(ShaftSpeedRefMax)
  ShaftSpeedMotor/1 -> Subsystem1/1(ShaftSpeed), Subsystem/2(shaftSpeedMotor)
  SpeedControllerReset/1 -> Subsystem/3(Reset)
  Switch/1 -> ContolTorque/1
  DeadBandController/1 -> Switch/2
  Subsystem1/1(ControlTorque) -> Rate Limiter/1
  Subsystem/1(ContolTorque) -> Switch/3
  Rate Limiter/1 -> Switch/1
  shaftSpeedRefMin/1 -> Rate Limiter1/1
  Rate Limiter1/1 -> Subsystem1/3(ShaftSpeedRefMin)

== system windEmulatorStep4/hptoSim/hptoModel/ControlAlgorithm/PressureBelowPmin/TorqueControl1 ==
  ActualTorqueInput : Inport
  TorqueRef : Inport  Port=2
  Pressure : Inport  Port=3
  Add : Sum
  Add1 : Sum
  Discrete-Time Integrator : DiscreteIntegrator  SampleTime=-1  ICPrevOutput=DiscIntNeverNeededParam  ICPrevScaledInput=DiscIntNeverNeededParam
  Divide : Product  Inputs=*/
  Gain : Gain  Gain=TorqueInputControl.PG
  Gain1 : Gain  Gain=TorqueInputControl.IG
  Gain2 : Gain  Gain=-1
  Product : Product
  Saturation : Saturate  UpperLimit=1  LowerLimit=-1
  Sum : Sum  Inputs=|-+
  UnitsConversion : Constant  Value=(100^3)*(2*pi)/(Dm_max*6894.75)
  ControlSignal1 : Outport
  wires:
  ActualTorqueInput/1 -> Sum/2
  Gain/1 -> Add/1
  Discrete-Time Integrator/1 -> Gain1/1
  Sum/1 -> Discrete-Time Integrator/1, Gain/1
  TorqueRef/1 -> Gain2/1, Sum/1
  Gain1/1 -> Add/2
  Saturation/1 -> ControlSignal1/1
  Add/1 -> Add1/1
  Add1/1 -> Saturation/1
  Pressure/1 -> Divide/2
  Divide/1 -> Product/1
  Product/1 -> Add1/2
  UnitsConversion/1 -> Product/2
  Gain2/1 -> Divide/1

== system windEmulatorStep4/hptoSim/hptoModel/HPTO/LinearVelInput/Subsystem ==
  Bus Creator : BusCreator  Inputs=3
  Ideal Force Sensor : fl_lib/Mechanical/Mechanical Sensors/Ideal Force Sensor
  Ideal Translational Motion Sensor : fl_lib/Mechanical/Mechanical Sensors/Ideal Translational Motion Sensor  reference=foundation.enum.MeasurementReference.difference  acceleration_port=false  velocity_port=true  position_port=true  offset=0 m
  Mechanical Translational Reference1 : fl_lib/Mechanical/Translational Elements/Mechanical Translational Reference
  PS-Simulink Converter : nesl_utility/PS-Simulink Converter  PhysicalDomain=network_engine_domain  SubClassName=ps_output  LeftPortType=input  RightPortType=output  PseudoPeriodic=off  Frequencies=[]  VectorFormat=1-D array  Unit=inherit  AffineConversion=off
  PS-Simulink Converter1 : nesl_utility/PS-Simulink Converter  PhysicalDomain=network_engine_domain  SubClassName=ps_output  LeftPortType=input  RightPortType=output  PseudoPeriodic=off  Frequencies=[]  VectorFormat=1-D array  Unit=inherit  AffineConversion=off
  PS-Simulink Converter2 : nesl_utility/PS-Simulink Converter  PhysicalDomain=network_engine_domain  SubClassName=ps_output  LeftPortType=input  RightPortType=output  PseudoPeriodic=off  Frequencies=[]  VectorFormat=1-D array  Unit=inherit  AffineConversion=off
  1 : PMIOPort  Side=Left
  2 : PMIOPort  Port=2  Side=Right
  LinearInput : Outport
  wires:
  PS-Simulink Converter/1 -> Bus Creator/3  "LinearPositionInput"
  PS-Simulink Converter1/1 -> Bus Creator/1  "ForceInput"
  PS-Simulink Converter2/1 -> Bus Creator/2  "LinearSpeedInput"
  Bus Creator/1 -> LinearInput/1
  connections:
  Mechanical Translational Reference1/LConn1 -- Ideal Translational Motion Sensor/RConn1
  2/RConn1 -- Ideal Force Sensor/LConn1 -- Ideal Translational Motion Sensor/LConn1
  PS-Simulink Converter/LConn1 -- Ideal Translational Motion Sensor/RConn3
  PS-Simulink Converter2/LConn1 -- Ideal Translational Motion Sensor/RConn2
  Ideal Force Sensor/RConn1 -- 1/RConn1
  Ideal Force Sensor/RConn2 -- PS-Simulink Converter1/LConn1

== system windEmulatorStep4/hptoSim/hptoModel/HPTO/LinearVelInput/WavebotModel ==
  PTOForce : Inport
  Fexc : Inport  Port=2
  Ideal Translational Velocity Source : fl_lib/Mechanical/Mechanical Sources/Ideal Translational Velocity Source
  Mechanical Translational Reference3 : fl_lib/Mechanical/Translational Elements/Mechanical Translational Reference
  Simulink-PS Converter : nesl_utility/Simulink-PS Converter  PhysicalDomain=network_engine_domain  SubClassName=ps_input  LeftPortType=input  RightPortType=output  PseudoPeriodic=off  Frequencies=[]  NoiseDistribution=none  NoiseParameters=[]  Unit=1  AffineConversion=off  FilteringAndDerivatives=provide  SimscapeFilterOrder=1  InputFilterTimeConstant=0.001  UdotUserProvided=0
  Sum : Sum  Inputs=|++
  WaveBotTF : cstblocks/LTI System  sys=Yi  IC=[]  PadeOrder=0
  VelSource : PMIOPort  Side=Right
  wires:
  PTOForce/1 -> Sum/2  "PTOForce"
  Fexc/1 -> Sum/1  "Fexc"
  WaveBotTF/1 -> Simulink-PS Converter/1  "vel"
  Sum/1 -> WaveBotTF/1
  connections:
  Ideal Translational Velocity Source/RConn1 -- Simulink-PS Converter/RConn1
  Mechanical Translational Reference3/LConn1 -- Ideal Translational Velocity Source/RConn2
  Ideal Translational Velocity Source/LConn1 -- VelSource/RConn1
